simulink model "bai_1"  (R2023a)
settings: Solver=VariableStepAuto  StartTime=0.0  StopTime=10.0  RelTol=1e-3
libraries: dspfdesign x2, simulink_extras x2, dspsrcs4 x2
settings Model: Creator=Admin  LastModifiedBy=Admin

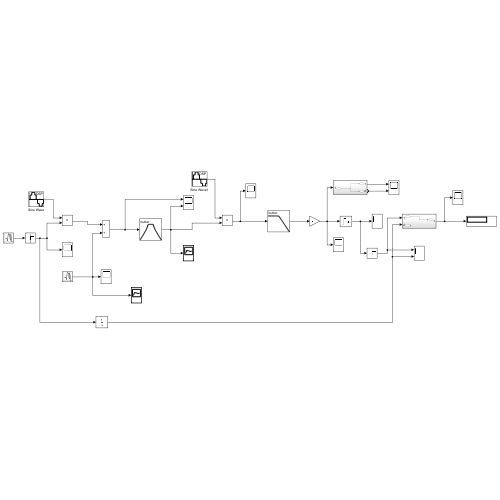
[thumbnail: Simulink's stored preview of the top-level diagram]
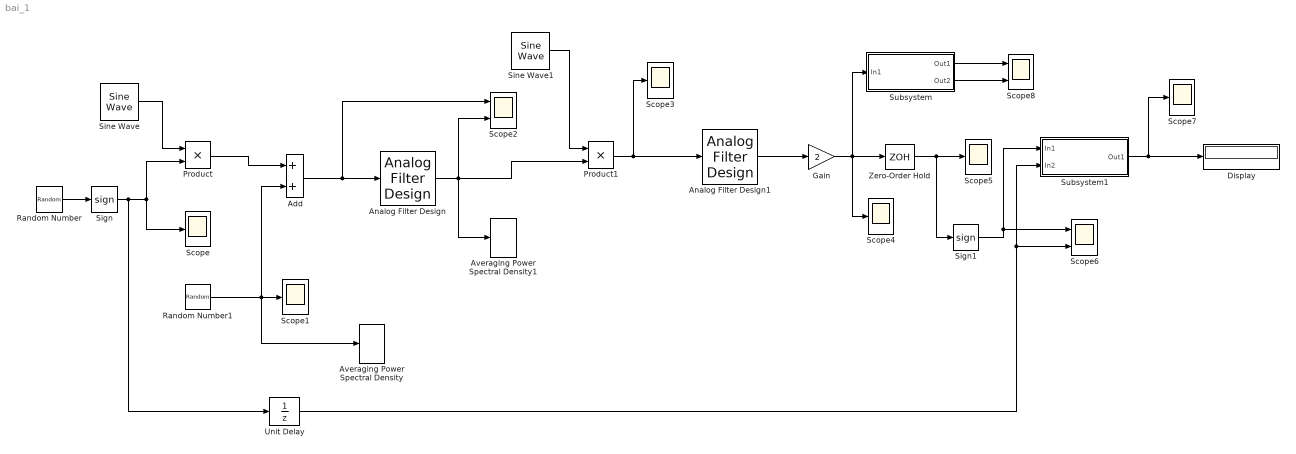
== system bai_1 ==
  Add : Sum
  Analog Filter Design : dspfdesign/Analog Filter Design  method=Butterworth  filttype=Bandpass  N=8  Wlo=30  Whi=80  Rp=2  Rs=40
  Analog Filter Design1 : dspfdesign/Analog Filter Design  method=Butterworth  filttype=Lowpass  N=8  Wlo=30  Whi=80  Rp=2  Rs=40
  Averaging Power Spectral Density : simulink_extras/Additional Sinks/Averaging Power Spectral Density  npts=128  fftpts=512  HowOften=64  sampleT=0.1
  Averaging Power Spectral Density1 : simulink_extras/Additional Sinks/Averaging Power Spectral Density  npts=128  fftpts=512  HowOften=64  sampleT=0.1
  Display : Display
  Gain : Gain  Gain=2
  Product : Product
  Product1 : Product
  Random Number : RandomNumber  SampleTime=0.1
  Random Number1 : RandomNumber  SampleTime=0.1
  Scope{,1,3..5,7} (6 alike) : Scope
  Scope2 : Scope  NumInputPorts=2
  Scope6 : Scope  NumInputPorts=2
  Scope8 : Scope  NumInputPorts=2
  Sign : Signum
  Sign1 : Signum
  Sine Wave : dspsrcs4/Sine Wave  Amplitude=1  Frequency=100  Phase=0  SampleMode=Discrete  OutComplex=Real  CompMethod=Trigonometric fcn  TableSize=Speed  SampleTime=1/1000  SamplesPerFrame=1  ResetState=Restart at time zero  OutputFrames=off  dataType=double  wordLen=16  udDataType=sfix(16)  fracBitsMode=Best precision  numFracBits=15  OutDataTypeStr=double  LastOutDataTypeStr=double
  Sine Wave1 : dspsrcs4/Sine Wave  Amplitude=1  Frequency=100  Phase=0  SampleMode=Discrete  OutComplex=Real  CompMethod=Trigonometric fcn  TableSize=Speed  SampleTime=1/1000  SamplesPerFrame=1  ResetState=Restart at time zero  OutputFrames=off  dataType=double  wordLen=16  udDataType=sfix(16)  fracBitsMode=Best precision  numFracBits=15  OutDataTypeStr=double  LastOutDataTypeStr=double
  Subsystem : Subsystem
  Subsystem1 : Subsystem
  Unit Delay : UnitDelay  SampleTime=-1  HasFrameUpgradeWarning=on
  Zero-Order Hold : ZeroOrderHold  SampleTime=-1
  wires:
  Sine Wave/1 -> Product/1
  Random Number/1 -> Sign/1
  Product/1 -> Add/1
  Random Number1/1 -> Averaging Power Spectral Density/1, Add/2, Scope1/1
  Sign/1 -> Unit Delay/1, Product/2, Scope/1
  Add/1 -> Scope2/1, Analog Filter Design/1
  Sine Wave1/1 -> Product1/1
  Analog Filter Design/1 -> Averaging Power Spectral Density1/1, Scope2/2, Product1/2
  Product1/1 -> Scope3/1, Analog Filter Design1/1
  Analog Filter Design1/1 -> Gain/1
  Gain/1 -> Scope4/1, Subsystem/1(In1), Zero-Order Hold/1
  Zero-Order Hold/1 -> Sign1/1, Scope5/1
  Unit Delay/1 -> Scope6/2, Subsystem1/2(In2)
  Sign1/1 -> Scope6/1, Subsystem1/1(In1)
  Subsystem1/1(Out1) -> Scope7/1, Display/1
  Subsystem/2(Out2) -> Scope8/2
  Subsystem/1(Out1) -> Scope8/1

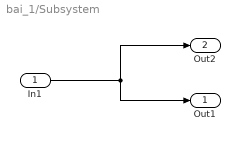
== system bai_1/Subsystem ==
  In1 : Inport
  Out1 : Outport
  Out2 : Outport  Port=2
  wires:
  In1/1 -> Out2/1, Out1/1

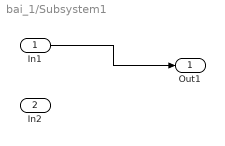
== system bai_1/Subsystem1 ==
  In1 : Inport
  In2 : Inport  Port=2
  Out1 : Outport
  wires:
  In1/1 -> Out1/1
